simulink library "testLibDW"  (R2015a)
settings: Solver=ode45  StartTime=0.0  StopTime=10.0  RelTol=1e-3
settings Model: Creator=shawn  LastModifiedBy=shawn

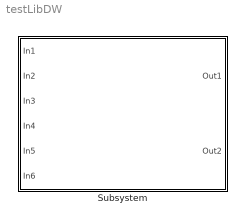
== system testLibDW ==
  Subsystem : Subsystem

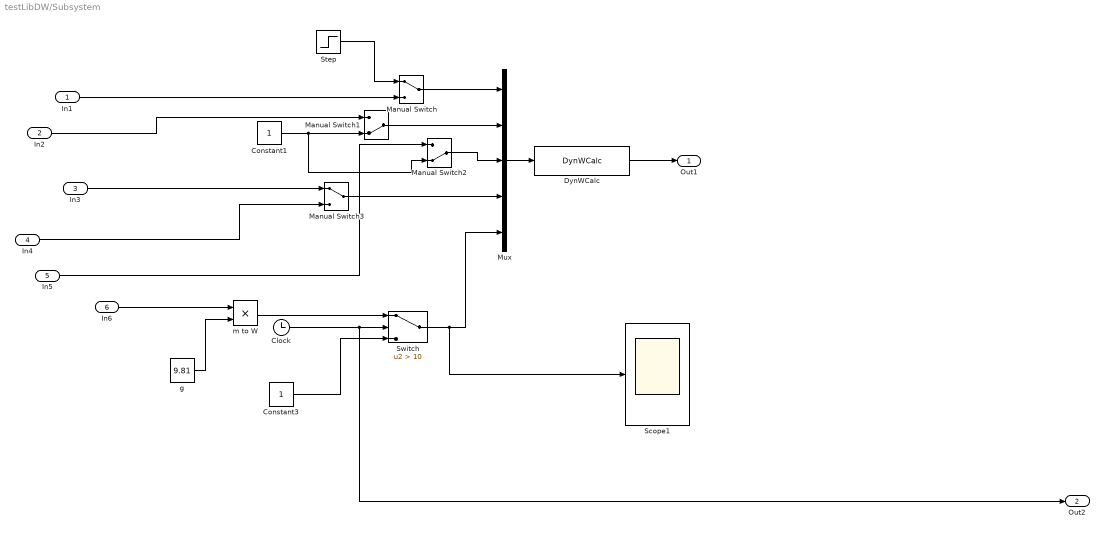
== system testLibDW/Subsystem ==
  In1 : Inport
  In2 : Inport  Port=2
  In3 : Inport  Port=3
  In4 : Inport  Port=4
  In5 : Inport  Port=5
  In6 : Inport  Port=6
  Clock : Clock
  Constant1 : Constant
  Constant3 : Constant
  DynWCalc : MATLABFcn  MATLABFcn=DynWCalc
      mask Display: disp('DynWCalc')
  Manual Switch : ManualSwitch
  Manual Switch1 : ManualSwitch  CurrentSetting=0
  Manual Switch2 : ManualSwitch  CurrentSetting=0
  Manual Switch3 : ManualSwitch
  Mux : Mux  Inputs=5
  Scope1 : Scope
  Step : Step  SampleTime=0
  Switch : Switch  Criteria=u2 > Threshold  Threshold=10
  g : Constant  Value=9.81
  m to W : Product
  Out1 : Outport
  Out2 : Outport  Port=2
  wires:
  Step/1 -> Manual Switch/1
  DynWCalc/1 -> Out1/1
  Manual Switch2/1 -> Mux/3
  Constant1/1 -> Manual Switch2/2, Manual Switch1/2
  Manual Switch3/1 -> Mux/4
  In3/1 -> Manual Switch3/1
  In5/1 -> Manual Switch2/1
  In1/1 -> Manual Switch/2
  In6/1 -> m to W/1
  Manual Switch/1 -> Mux/1
  g/1 -> m to W/2
  Switch/1 -> Scope1/1, Mux/5
  Mux/1 -> DynWCalc/1
  In4/1 -> Manual Switch3/2
  m to W/1 -> Switch/1
  In2/1 -> Manual Switch1/1
  Constant3/1 -> Switch/3
  Clock/1 -> Out2/1, Switch/2
  Manual Switch1/1 -> Mux/2
